simulink model "PD1_DCS_810698349"  (R2021b)
settings: Solver=VariableStepAuto  StartTime=0.0  StopTime=3  FixedStep=0.00001*Ts  RelTol=1e-3
undefined symbols (not defined in the file): Ad, C, g, G, H, K, Kc, L, Lo, M, N, R, Ts, wd, y0, y00
settings Model: Creator=SinaK  LastModifiedBy=SinaK

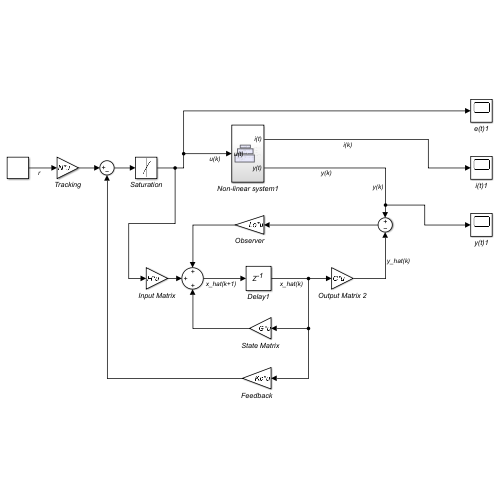
[thumbnail: Simulink's stored preview of the top-level diagram]
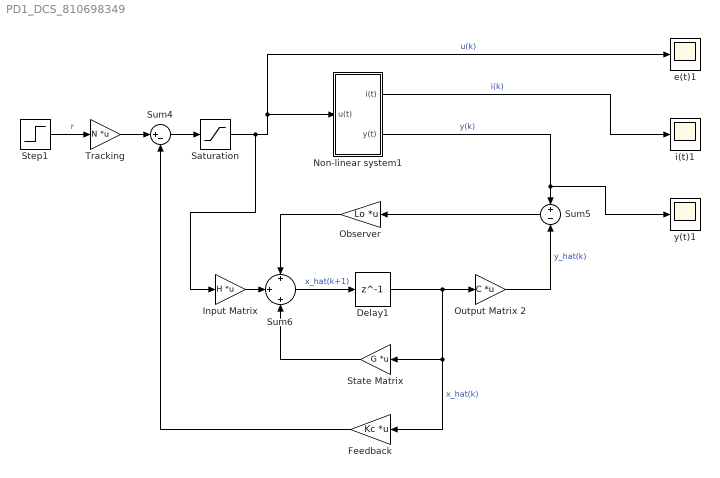
== system PD1_DCS_810698349 ==
  Delay1 : Delay  DelayLength=1  SampleTime=Ts
  Feedback : Gain  Gain=Kc  Multiplication=Matrix(K*u)
  Input Matrix : Gain  Gain=H  Multiplication=Matrix(K*u)
  Non-linear system1 : Subsystem
  Observer : Gain  Gain=Lo  Multiplication=Matrix(K*u)
  Output Matrix 2 : Gain  Gain=C  Multiplication=Matrix(K*u)
  Saturation : Saturate  UpperLimit=12  LowerLimit=0
  State Matrix : Gain  Gain=G  Multiplication=Matrix(K*u)
  Step1 : Step  Time=0  After=y0  SampleTime=Ts
  Sum4 : Sum  Inputs=|+-
  Sum5 : Sum  Inputs=+|-
  Sum6 : Sum  Inputs=+|+|+
  Tracking : Gain  Gain=N  Multiplication=Matrix(K*u)
  e(t)1 : Scope
  i(t)1 : Scope
  y(t)1 : Scope
  wires:
  Tracking/1 -> Sum4/1
  Saturation/1 -> Input Matrix/1, Non-linear system1/1(u(t)), e(t)1/1  "u(k)"
  Sum4/1 -> Saturation/1
  Sum6/1 -> Delay1/1  "x_hat(k+1)"
  Input Matrix/1 -> Sum6/2
  Output Matrix 2/1 -> Sum5/2  "y_hat(k)"
  Sum5/1 -> Observer/1
  Delay1/1 -> Output Matrix 2/1, Feedback/1, State Matrix/1  "x_hat(k)"
  Non-linear system1/1(i(t)) -> i(t)1/1  "i(k)"
  Observer/1 -> Sum6/1
  Feedback/1 -> Sum4/2
  State Matrix/1 -> Sum6/3
  Step1/1 -> Tracking/1  "r"
  Non-linear system1/2(y(t)) -> y(t)1/1, Sum5/1  "y(k)"

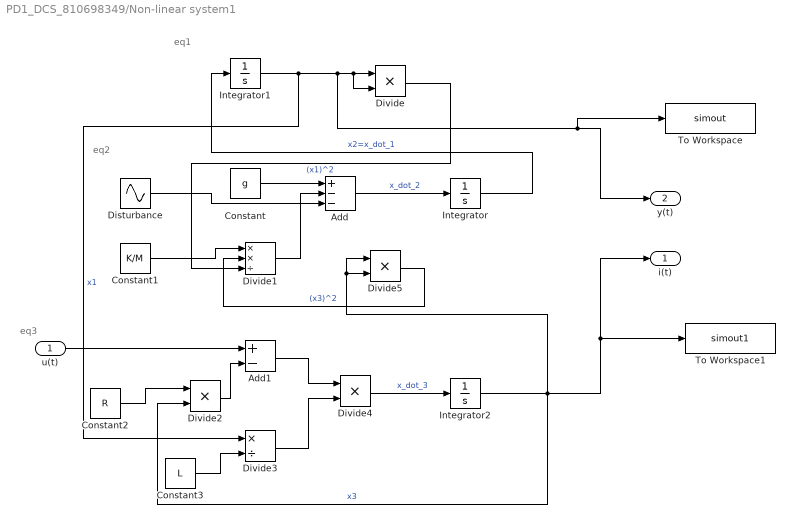
== system PD1_DCS_810698349/Non-linear system1 ==
  note: eq1
  note: eq2
  note: eq3
  u(t) : Inport
  Add : Sum  Inputs=+--
  Add1 : Sum  Inputs=+-
  Constant : Constant  Value=g  SampleTime=Ts
  Constant1 : Constant  Value=K/M  SampleTime=Ts
  Constant2 : Constant  Value=R  SampleTime=Ts
  Constant3 : Constant  Value=L  SampleTime=Ts
  Disturbance : Sin  Amplitude=Ad/M  Frequency=wd  SampleTime=Ts
  Divide{,2,4..5} (4 alike) : Product  Inputs=**
  Divide1 : Product  Inputs=**/
  Divide3 : Product  Inputs=*/
  Integrator : Integrator
  Integrator1 : Integrator  InitialCondition=y00
  Integrator2 : Integrator
  To Workspace : ToWorkspace  VariableName=simout  SaveFormat=Timeseries  SampleTime=-1
      settings: Decimation=3
  To Workspace1 : ToWorkspace  VariableName=simout1  SaveFormat=Timeseries  SampleTime=-1
      settings: Decimation=3
  i(t) : Outport
  y(t) : Outport  Port=2
  wires:
  Add/1 -> Integrator/1  "x_dot_2"
  Divide/1 -> Divide1/3  "(x1)^2"
  Integrator/1 -> Integrator1/1  "x2=x_dot_1"
  Integrator2/1 -> i(t)/1, To Workspace1/1, Divide5/1, Divide5/2, Divide2/2  "x3"
  Divide1/1 -> Add/2
  Add1/1 -> Divide4/1
  Constant3/1 -> Divide3/2
  Constant2/1 -> Divide2/1
  Divide5/1 -> Divide1/2  "(x3)^2"
  Integrator1/1 -> Divide3/1, To Workspace/1, y(t)/1, Divide/2, Divide/1  "x1"
  Divide4/1 -> Integrator2/1  "x_dot_3"
  Constant1/1 -> Divide1/1
  Constant/1 -> Add/1
  Divide3/1 -> Divide4/2
  Divide2/1 -> Add1/2
  u(t)/1 -> Add1/1
  Disturbance/1 -> Add/3
